simulink model "TestWCPS_v1"  (R2018a)
settings: Solver=VariableStepAuto  StartTime=0.0  StopTime=1000  RelTol=1e-3
values from neighbouring files (symbols this model uses):
  A = [1.38 -0.2077 6.715 -5.676;-0.5814 -4.29 0 0.675;1.067 4.273 -6.654 5.893;0.048 4.273 1.343 -2.104]    [NCS_code.m]
  Ac = [0 0;0 0]    [NCS_code.m]
  B = [0 0;5.679 0;1.136 -3.146;1.136 0]    [NCS_code.m]
  Bc = [0 1;1 0]    [NCS_code.m]
  C = [1 0 1 -1;0 1 0 0]    [NCS_code.m]
  Cc = [2 0;0 -8]    [NCS_code.m]
  D = [0 0;0 0]    [NCS_code.m]
  Dc = [0 2;-5 0]    [NCS_code.m]
  delta_t_moter = 10    [NCS_code.m]
libraries: simulink x1
settings Model: Creator=root  LastModifiedBy=root

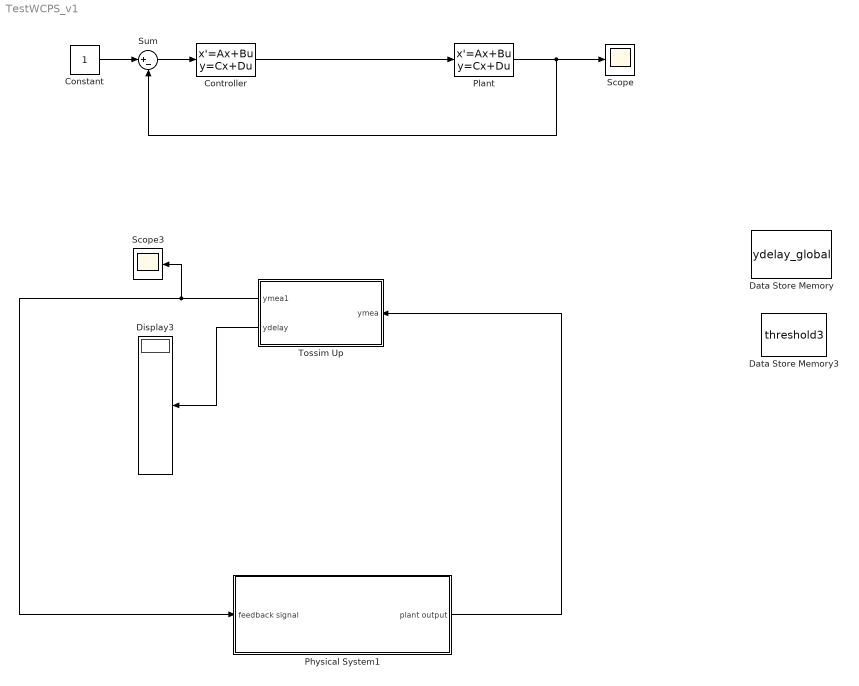
== system TestWCPS_v1 ==
  Constant : Constant
  Controller : StateSpace  A=Ac  B=Bc  C=Cc  D=Dc  InitialCondition=0
  Data Store Memory : DataStoreMemory  DataStoreName=ydelay_global  ReadBeforeWriteMsg=warning  WriteAfterWriteMsg=warning  WriteAfterReadMsg=warning  InitialValue=[1; 1; 1; 1; 1; 1; 1; 1; 1; 1; 1; 1; 1; 1; 1]  ShowAdditionalParam=off  OutDataTypeStr=uint32
  Data Store Memory3 : DataStoreMemory  DataStoreName=threshold3  ReadBeforeWriteMsg=warning  WriteAfterWriteMsg=warning  WriteAfterReadMsg=warning  InitialValue=th3_initial  ShowAdditionalParam=off  OutDataTypeStr=double
  Display3 : Display
  "Physical System1 " : Subsystem
  Plant : StateSpace  A=A  B=B  C=C  D=D  InitialCondition=0
  Scope : Scope
  Scope3 : Scope
  Sum : Sum  Inputs=|+-
  Tossim Up : MATLAB Function  TreatAsAtomicUnit=on
  wires:
  Plant/1 -> Sum/2, Scope/1
  Controller/1 -> Plant/1
  Sum/1 -> Controller/1
  Constant/1 -> Sum/1
  Tossim Up/2(ydelay) -> Display3/1
  Tossim Up/1(ymea1) -> "Physical System1 "/1("feedback signal "), Scope3/1
  "Physical System1 "/1("plant output ") -> Tossim Up/1(ymea)

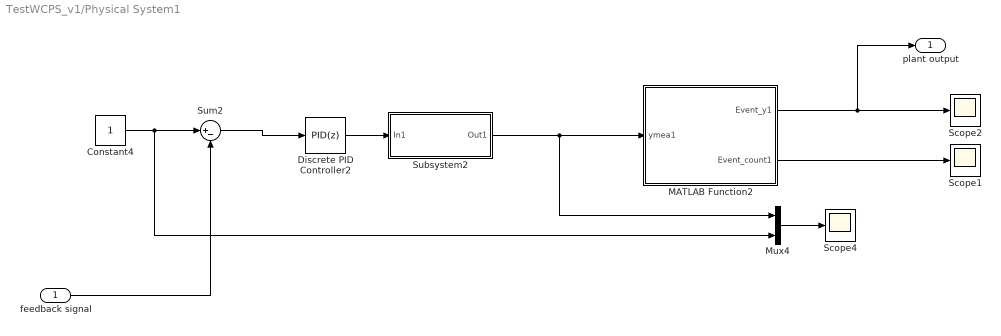
== system TestWCPS_v1/Physical System1  ==
  "feedback signal " : Inport
  Constant4 : Constant
  Discrete PID Controller2 : simulink/Continuous/PID Controller  Controller=PID  TimeDomain=Discrete-time  SampleTime=delta_t_moter  IntegratorMethod=Forward Euler  FilterMethod=Forward Euler  Form=Parallel  UseFilter=on  ControllerParametersSource=internal  P=0.0705520945054552  I=0.014110418901091  D=0  N=100  InitialConditionSource=internal  InitialConditionForIntegrator=0  InitialConditionForFilter=0  ExternalReset=none  LimitOutput=off  UpperSaturationLimit=inf  LowerSaturationLimit=-inf  LinearizeAsGain=off  AntiWindupMode=none  Kb=1  TrackingMode=off  Kt=1  PParamMin=[]  PParamMax=[]  IParamMin=[]  IParamMax=[]  DParamMin=[]  DParamMax=[]  NParamMin=[]  NParamMax=[]  KbParamMin=[]  KbParamMax=[]  KtParamMin=[]  KtParamMax=[]  POutMin=[]  POutMax=[]  IOutMin=[]  IOutMax=[]  DOutMin=[]  DOutMax=[]  NOutMin=[]  NOutMax=[]  KbOutMin=[]  KbOutMax=[]  KtOutMin=[]  KtOutMax=[]  IntegratorOutMin=[]  IntegratorOutMax=[]  FilterOutMin=[]  FilterOutMax=[]  SumOutMin=[]  SumOutMax=[]  SumI1OutMin=[]  SumI1OutMax=[]  SumI2OutMin=[]  SumI2OutMax=[]  SumI3OutMin=[]  SumI3OutMax=[]  SumDOutMin=[]  SumDOutMax=[]  SaturationOutMin=[]  SaturationOutMax=[]  IntegratorContinuousStateAttributes=''  IntegratorStateMustResolveToSignalObject=off  IntegratorRTWStateStorageClass=Auto  FilterContinuousStateAttributes=''  FilterStateMustResolveToSignalObject=off  FilterRTWStateStorageClass=Auto  DifferentiatorICPrevScaledInput=0  DifferentiatorOutMin=[]  DifferentiatorOutMax=[]  FilterDiffOutCoefMin=[]  FilterDiffOutCoefMax=[]  SumDenOutMin=[]  SumDenOutMax=[]  SumNumOutMin=[]  SumNumOutMax=[]  ReciprocalOutMin=[]  ReciprocalOutMax=[]  DivideOutMin=[]  DivideOutMax=[]  TunerSelectOption=Transfer Function Based (PID Tuner App)
  MATLAB Function2 : MATLAB Function  TreatAsAtomicUnit=on
  Mux4 : Mux  Inputs=2
  Scope1 : Scope
  Scope2 : Scope
  Scope4 : Scope
  Subsystem2 : Subsystem
  Sum2 : Sum  Inputs=|+-
  "plant output " : Outport
  wires:
  Discrete PID Controller2/1 -> Subsystem2/1(In1)
  MATLAB Function2/1(Event_y1) -> "plant output "/1, Scope2/1
  MATLAB Function2/2(Event_count1) -> Scope1/1
  Subsystem2/1(Out1) -> MATLAB Function2/1(ymea1), Mux4/1
  Mux4/1 -> Scope4/1
  Constant4/1 -> Mux4/2, Sum2/1
  Sum2/1 -> Discrete PID Controller2/1
  "feedback signal "/1 -> Sum2/2

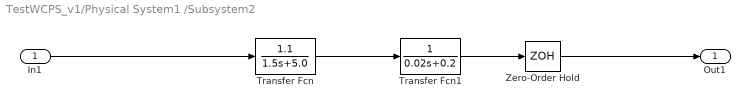
== system TestWCPS_v1/Physical System1 /Subsystem2 ==
  In1 : Inport
  Transfer Fcn : TransferFcn  Numerator=[1.1]  Denominator=[1.5 5.0]
  Transfer Fcn1 : TransferFcn  Denominator=[0.02 0.2]
  Zero-Order Hold : ZeroOrderHold  SampleTime=delta_t_moter
  Out1 : Outport
  wires:
  Transfer Fcn/1 -> Transfer Fcn1/1
  In1/1 -> Transfer Fcn/1
  Transfer Fcn1/1 -> Zero-Order Hold/1
  Zero-Order Hold/1 -> Out1/1

== matlab function TestWCPS_v1/Tossim Up ==
  settings: updateMethod=DISCRETE
  data: ymea1 output; ymea input; ydelay output; ydelay_global data_store_memory
function [ymea1, ydelay]  = Tossim_block(ymea)
% Inputs:
% ymea: measurement from structure
% Outputs:
% ymea1: measurement output
% ydelay: delay traces
persistent delay1 past_ymea % delay trace
persistent i Task_period % count
global ydelay_global


% allow these matlab functions to be used in Embedded Matlab block
eml.extrinsic('python');
eml.extrinsic('num2str');
eml.extrinsic('str2num');
eml.extrinsic('delay_summary');
eml.extrinsic('disp');
eml.extrinsic('ps_aggregation');
eml.extrinsic('for');
eml.extrinsic('end');

if isempty(i)
    i = 0;
    past_ymea = ymea;
    Task_period = [10 10 8];        %Task_period=[10 10 4] * 10
end

ydelay = [1 0 0 0 0 0 0 0 0]';
% call python to communicate with TOSSIM

call_count = 1; %Superframelength
rssi = -69;%sensor rssi

%Transfer Event count to TOSSIM
Event_count1 = 11;
Event_count2 = 12;
[resultz] = ps_aggregation(call_count, rssi, Event_count1, Event_count2);%here call TOSSIM Client ----yh
%resultz = [1, 0, 0, 0, 0, 0, 0, 0]; 
    
end_to_end_delivery_result_aggregated = sum(resultz);

resultz

%[delay] = delay_summary(end_to_end_delivery_result_aggregated);
[delay] = delay_summary(resultz);

delay;

% for event trigger!!!
Task_period_time = Task_period * 10;

ydelay = delay';

delay1 = ydelay;
x =ydelay(2);
i = i+1;

%ymea1 = ymea;

for i_yg = 1:9
    ydelay_global(i_yg, 1) = ydelay(i_yg, 1);
end

delay = ydelay';


ymea_v1_index = 1;


if delay(1,ymea_v1_index + 1)~=88
    ans1 = past_ymea;
    %ymea1 = new_trans_ymea;
    past_ymea = ymea;
else
    ans1 = past_ymea;
end

ymea1 = ans1;

== matlab function TestWCPS_v1/Physical System1 /MATLAB Function2 ==
  data: ymea1 input; Event_y1 output; threshold3 data_store_memory; Event_count1 output
function [Event_y1, Event_count1] = event_trigger1(ymea1)

persistent previous_ymea tmp_eventcount
persistent i %count
global threshold3


if isempty(i)
    i = 0;
    tmp_eventcount = 0;
    previous_ymea = 0;
end

compare = abs(ymea1 - previous_ymea);
if (compare) >= threshold3
    ans = ymea1;
    previous_ymea = ymea1;
    tmp_eventcount = tmp_eventcount + 1;
else
    ans = previous_ymea;
end

i = i + 1;
Event_count1 = tmp_eventcount;
Event_y1 = ans;
